simulink model "RateLimit2020"  (R2015a)
settings: Solver=ode45  StartTime=0.0  StopTime=60  RelTol=1e-3
libraries: dspvision x3, dspsnks4 x1
settings Model: Creator=ekulasek  LastModifiedBy=ekulasek

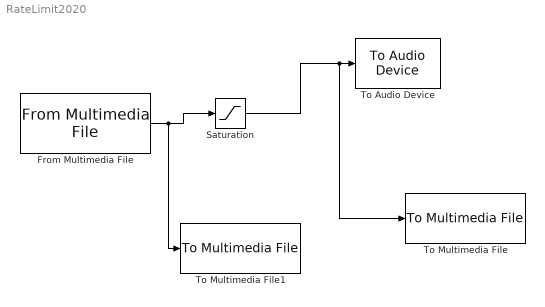
== system RateLimit2020 ==
  From Multimedia File : dspvision/From Multimedia File  inputFilename=/home/ekulasek/Malabe/classes/SignalsAndSystems/Programs/Adaraneeya_Wassanaya.wav  loop=on  numPlays=inf  outputStreams=Audio only  videoDataType=single  audioDataType=double  inheritSampleTime=on  userDefinedSampleTime=1/30  noAudioOutput=off  isIntensityVideo=off  fourcc=RGB  colorVideoFormat=Separate color signals  outputEOF=off  dataOrg=Column-major  audioFrameSize=1024  computeAudioFrameSize=off  outSamplingMode=Sample based
  Saturation : Saturate  UpperLimit=0.05  LowerLimit=-0.05
  To Audio Device : dspsnks4/To Audio Device  deviceName=Default  inheritSampleRate=on  sampleRate=44100  deviceDatatype=Determine from input data type  autoBufferSize=on  bufferSize=4096  queueDuration=1.0  defaultOutputChannelMapping=on  outputChannelMapping=1:2  outputNumUnderrunSamples=off
  To Multimedia File : dspvision/To Multimedia File  outputFilename=/home/ekulasek/Malabe/classes/SignalsAndSystems/Programs/cut07.wav  streamSelection=Audio only  videoCompressor=None (uncompressed)  audioCompressor=None (uncompressed)  imagePorts=Separate color signals  fileType=WAV  audioDatatype=16-bit integer  fourcc=RGB  videoQuality=75  mj2000CompFactor=10
  To Multimedia File1 : dspvision/To Multimedia File  outputFilename=/home/ekulasek/Malabe/classes/SignalsAndSystems/Programs/cut06.wav  streamSelection=Audio only  videoCompressor=None (uncompressed)  audioCompressor=None (uncompressed)  imagePorts=Separate color signals  fileType=WAV  audioDatatype=16-bit integer  fourcc=RGB  videoQuality=75  mj2000CompFactor=10
  wires:
  From Multimedia File/1 -> To Multimedia File1/1, Saturation/1
  Saturation/1 -> To Multimedia File/1, To Audio Device/1
